simulink model "PthSet_TrqCalc"  (R2018a)
settings: configuration reference "cs_ert" (kept outside this file)
undefined symbols (not defined in the file): EngState, PthSet_trqOffs_C, TRQ_ZERO
libraries: simulink x4
settings Model: DataDictionary=PthSet_TrqCalc.sldd  Creator=zhoutinglin  LastModifiedBy=zhoutinglin

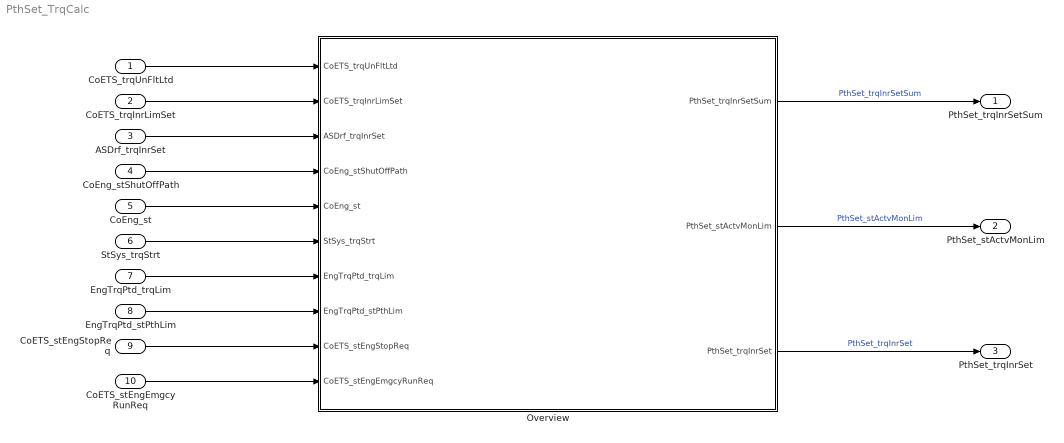
== system PthSet_TrqCalc ==
  CoETS_trqUnFltLtd : Inport  Description=Grip reliable exclude  OutMin=-3276  OutMax=3276  OutDataTypeStr=Torq  PortDimensions=[1 1]
  CoETS_trqInrLimSet : Inport  Description=Powertrain torque ratio  Port=2  OutMin=-3000  OutMax=3000  OutDataTypeStr=Torq  PortDimensions=[1 1]
  ASDrf_trqInrSet : Inport  Description=Limited idle speed governor torque  Port=3  OutMin=-3000  OutMax=3000  OutDataTypeStr=Torq  Unit=Nm  PortDimensions=[1 1]
  CoEng_stShutOffPath : Inport  Description=Limitation torque without the part of the speed governor  Port=4  OutMin=0  OutMax=65535  OutDataTypeStr=State2  PortDimensions=[1 1]
  CoEng_st : Inport  Description=ASD reference filter torque output  Port=5  OutDataTypeStr=Enum:EngState  PortDimensions=[1 1]
  StSys_trqStrt : Inport  Description=ASD disturbance compensator torque output  Port=6  OutMin=-3000  OutMax=3000  OutDataTypeStr=Torq  Unit=Nm  PortDimensions=[1 1]
  EngTrqPtd_trqLim : Inport  Description=Active shut-off paths resulting from active reversible,irreversible and afterrun shut-off paths  Port=7  OutMin=-3276  OutMax=3276  OutDataTypeStr=Torq  PortDimensions=[1 1]
  EngTrqPtd_stPthLim : Inport  Description=Engine coordinator state  Port=8  OutMin=0  OutMax=255  OutDataTypeStr=State  PortDimensions=[1 1]
  CoETS_stEngStopReq : Inport  Description=Engine starting torque  Port=9  OutMin=0  OutMax=1  OutDataTypeStr=boolean  PortDimensions=[1 1]
  CoETS_stEngEmgcyRunReq : Inport  Description=State of overrun detection (0: No overrun; 1: overrun)  Port=10  OutMin=0  OutMax=1  OutDataTypeStr=boolean  PortDimensions=[1 1]
  Overview : Subsystem
  PthSet_trqInrSetSum : Outport
  PthSet_stActvMonLim : Outport  Port=2
  PthSet_trqInrSet : Outport  Port=3
  wires:
  CoETS_trqUnFltLtd/1 -> Overview/1(CoETS_trqUnFltLtd)
  CoETS_trqInrLimSet/1 -> Overview/2(CoETS_trqInrLimSet)
  ASDrf_trqInrSet/1 -> Overview/3(ASDrf_trqInrSet)
  CoEng_stShutOffPath/1 -> Overview/4(CoEng_stShutOffPath)
  CoEng_st/1 -> Overview/5(CoEng_st)
  StSys_trqStrt/1 -> Overview/6(StSys_trqStrt)
  EngTrqPtd_trqLim/1 -> Overview/7(EngTrqPtd_trqLim)
  EngTrqPtd_stPthLim/1 -> Overview/8(EngTrqPtd_stPthLim)
  CoETS_stEngStopReq/1 -> Overview/9(CoETS_stEngStopReq)
  CoETS_stEngEmgcyRunReq/1 -> Overview/10(CoETS_stEngEmgcyRunReq)
  Overview/1(PthSet_trqInrSetSum) -> PthSet_trqInrSetSum/1  "PthSet_trqInrSetSum"
  Overview/2(PthSet_stActvMonLim) -> PthSet_stActvMonLim/1  "PthSet_stActvMonLim"
  Overview/3(PthSet_trqInrSet) -> PthSet_trqInrSet/1  "PthSet_trqInrSet"

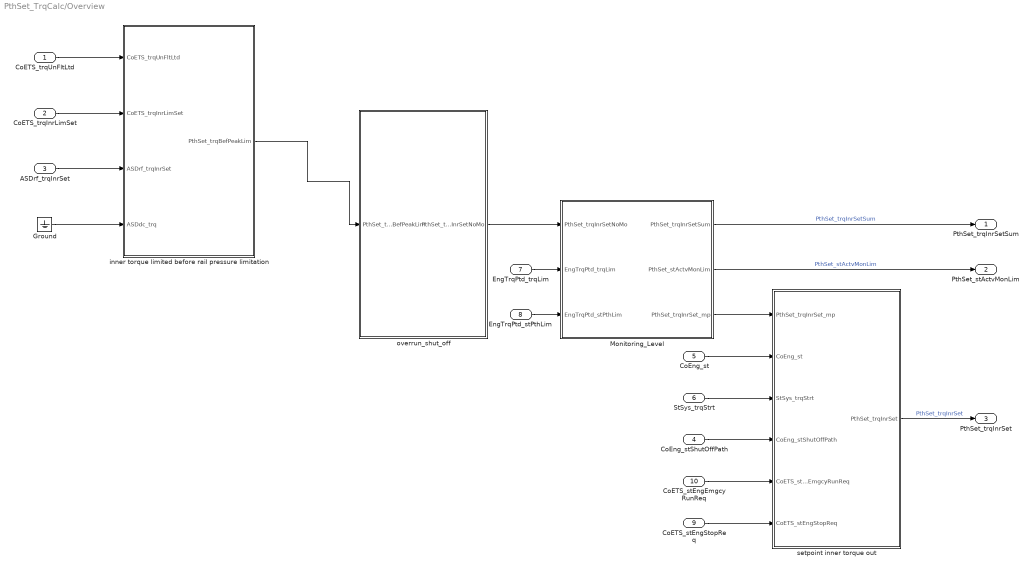
== system PthSet_TrqCalc/Overview ==
  CoETS_trqUnFltLtd : Inport  Tag=Nm
  CoETS_trqInrLimSet : Inport  Tag=Nm  Port=2
  ASDrf_trqInrSet : Inport  Tag=Nm  Port=3
  CoEng_stShutOffPath : Inport  Port=4
  CoEng_st : Inport  Port=5
  StSys_trqStrt : Inport  Tag=Nm  Port=6
  EngTrqPtd_trqLim : Inport  Tag=Nm  Port=7
  EngTrqPtd_stPthLim : Inport  Port=8
  CoETS_stEngStopReq : Inport  Port=9
  CoETS_stEngEmgcyRunReq : Inport  Port=10
  Ground : Ground
  Monitoring_Level : Subsystem
  inner torque limited before rail pressure limitation : Subsystem
  overrun_shut_off : Subsystem
  setpoint inner torque out : Subsystem
  PthSet_trqInrSetSum : Outport  Tag=Nm
  PthSet_stActvMonLim : Outport  Port=2
  PthSet_trqInrSet : Outport  Tag=Nm  Port=3
  wires:
  EngTrqPtd_trqLim/1 -> Monitoring_Level/2(EngTrqPtd_trqLim)
  CoETS_stEngStopReq/1 -> setpoint inner torque out/6(CoETS_stEngStopReq)
  inner torque limited before rail pressure limitation/1(PthSet_trqBefPeakLim) -> overrun_shut_off/1(PthSet_trqBefPeakLim)
  CoETS_trqInrLimSet/1 -> inner torque limited before rail pressure limitation/2(CoETS_trqInrLimSet)
  Monitoring_Level/3(PthSet_trqInrSet_mp) -> setpoint inner torque out/1(PthSet_trqInrSet_mp)
  Monitoring_Level/2(PthSet_stActvMonLim) -> PthSet_stActvMonLim/1  "PthSet_stActvMonLim"
  CoETS_trqUnFltLtd/1 -> inner torque limited before rail pressure limitation/1(CoETS_trqUnFltLtd)
  CoEng_stShutOffPath/1 -> setpoint inner torque out/4(CoEng_stShutOffPath)
  CoETS_stEngEmgcyRunReq/1 -> setpoint inner torque out/5(CoETS_stEngEmgcyRunReq)
  StSys_trqStrt/1 -> setpoint inner torque out/3(StSys_trqStrt)
  ASDrf_trqInrSet/1 -> inner torque limited before rail pressure limitation/3(ASDrf_trqInrSet)
  Monitoring_Level/1(PthSet_trqInrSetSum) -> PthSet_trqInrSetSum/1  "PthSet_trqInrSetSum"
  overrun_shut_off/1(PthSet_trqInrSetNoMo) -> Monitoring_Level/1(PthSet_trqInrSetNoMo)
  setpoint inner torque out/1(PthSet_trqInrSet) -> PthSet_trqInrSet/1  "PthSet_trqInrSet"
  CoEng_st/1 -> setpoint inner torque out/2(CoEng_st)
  Ground/1 -> inner torque limited before rail pressure limitation/4(ASDdc_trq)
  EngTrqPtd_stPthLim/1 -> Monitoring_Level/3(EngTrqPtd_stPthLim)

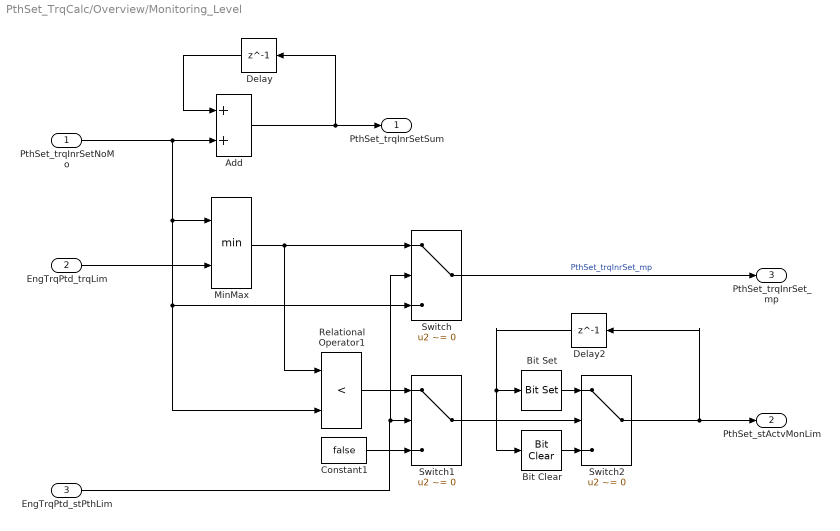
== system PthSet_TrqCalc/Overview/Monitoring_Level ==
  PthSet_trqInrSetNoMo : Inport
  EngTrqPtd_trqLim : Inport  Port=2
  EngTrqPtd_stPthLim : Inport  Port=3
  Add : Sum  SaturateOnIntegerOverflow=on  InputSameDT=on
  Bit Clear : simulink/Logic and Bit Operations/Bit Clear  iBit=0
      settings: SourceProductName=Simulink  SourceProductBaseCode=SL
  Bit Set : simulink/Logic and Bit Operations/Bit Set  iBit=0
      settings: SourceProductName=Simulink  SourceProductBaseCode=SL
  Constant1 : Constant  Value=false  OutDataTypeStr=Inherit: Inherit via back propagation
  Delay : Delay  DelayLength=1  InitialCondition=0
  Delay2 : Delay  DelayLength=1  InitialCondition=0
  MinMax : MinMax  Inputs=2  InputSameDT=on
  Relational Operator1 : RelationalOperator  Operator=<  OutDataTypeStr=boolean  RndMeth=Simplest  InputSameDT=on
  Switch : Switch  Criteria=u2 ~= 0  InputSameDT=on
  Switch1 : Switch  Criteria=u2 ~= 0  InputSameDT=on
  Switch2 : Switch  Criteria=u2 ~= 0  InputSameDT=on
  PthSet_trqInrSetSum : Outport
  PthSet_stActvMonLim : Outport  Port=2
  PthSet_trqInrSet_mp : Outport  Port=3
  wires:
  Delay2/1 -> Bit Set/1, Bit Clear/1
  Bit Clear/1 -> Switch2/3
  Bit Set/1 -> Switch2/1
  Switch2/1 -> PthSet_stActvMonLim/1, Delay2/1
  Switch1/1 -> Switch2/2
  Switch/1 -> PthSet_trqInrSet_mp/1  "PthSet_trqInrSet_mp"
  EngTrqPtd_stPthLim/1 -> Switch1/2, Switch/2
  Constant1/1 -> Switch1/3
  Relational Operator1/1 -> Switch1/1
  MinMax/1 -> Switch/1, Relational Operator1/1
  EngTrqPtd_trqLim/1 -> MinMax/2
  Delay/1 -> Add/1
  Add/1 -> PthSet_trqInrSetSum/1, Delay/1
  PthSet_trqInrSetNoMo/1 -> Add/2, MinMax/1, Switch/3, Relational Operator1/2

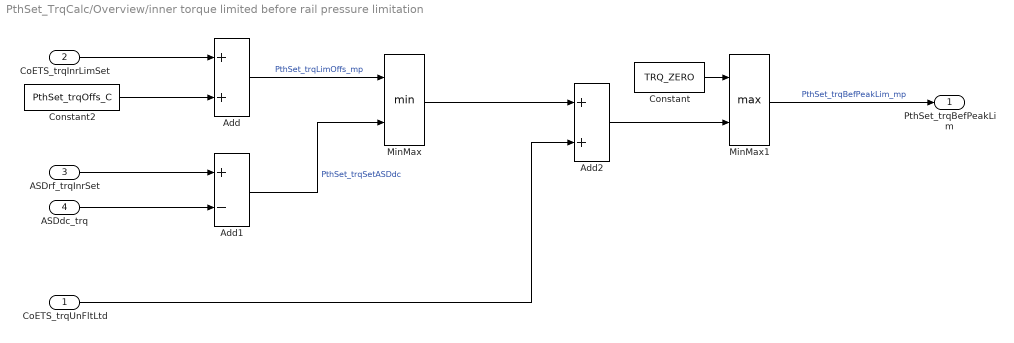
== system PthSet_TrqCalc/Overview/inner torque limited before rail pressure limitation ==
  CoETS_trqUnFltLtd : Inport
  CoETS_trqInrLimSet : Inport  Port=2
  ASDrf_trqInrSet : Inport  Port=3
  ASDdc_trq : Inport  Port=4
  Add : Sum  SaturateOnIntegerOverflow=on  InputSameDT=on
  Add1 : Sum  Inputs=+-  OutDataTypeStr=Inherit: Inherit via back propagation  SaturateOnIntegerOverflow=on  InputSameDT=on
  Add2 : Sum  SaturateOnIntegerOverflow=on  InputSameDT=on
  Constant : Constant  Value=TRQ_ZERO  OutDataTypeStr=Inherit: Inherit via back propagation
  Constant2 : Constant  Value=PthSet_trqOffs_C
  MinMax : MinMax  Inputs=2  InputSameDT=on
  MinMax1 : MinMax  Function=max  Inputs=2  InputSameDT=on
  PthSet_trqBefPeakLim : Outport
  wires:
  Constant2/1 -> Add/2
  ASDdc_trq/1 -> Add1/2
  Add2/1 -> MinMax1/2
  CoETS_trqInrLimSet/1 -> Add/1
  ASDrf_trqInrSet/1 -> Add1/1
  Add1/1 -> MinMax/2  "PthSet_trqSetASDdc"
  Add/1 -> MinMax/1  "PthSet_trqLimOffs_mp"
  CoETS_trqUnFltLtd/1 -> Add2/2
  MinMax/1 -> Add2/1
  Constant/1 -> MinMax1/1
  MinMax1/1 -> PthSet_trqBefPeakLim/1  "PthSet_trqBefPeakLim_mp"

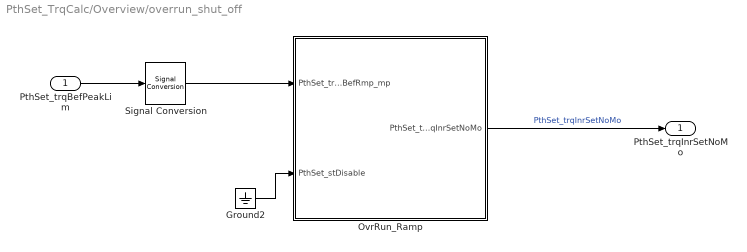
== system PthSet_TrqCalc/Overview/overrun_shut_off ==
  PthSet_trqBefPeakLim : Inport
  Ground2 : Ground
  OvrRun_Ramp : Subsystem
  Signal Conversion : SignalConversion  OverrideOpt=off
  PthSet_trqInrSetNoMo : Outport
  wires:
  PthSet_trqBefPeakLim/1 -> Signal Conversion/1
  Ground2/1 -> OvrRun_Ramp/2(PthSet_stDisable)
  OvrRun_Ramp/1(PthSet_trqInrSetNoMo) -> PthSet_trqInrSetNoMo/1  "PthSet_trqInrSetNoMo"
  Signal Conversion/1 -> OvrRun_Ramp/1(PthSet_trqBefRmp_mp)

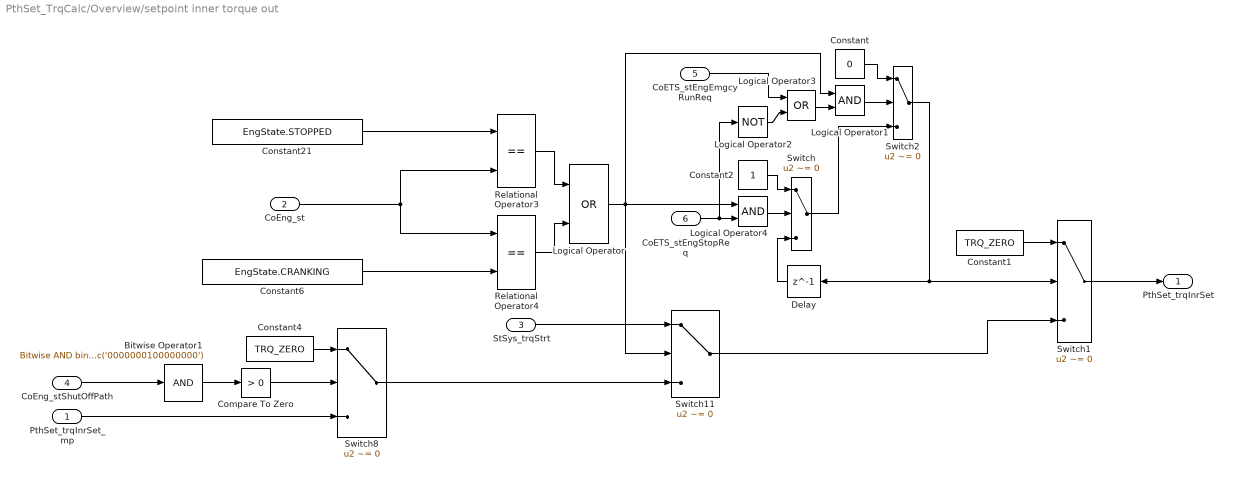
== system PthSet_TrqCalc/Overview/setpoint inner torque out ==
  PthSet_trqInrSet_mp : Inport
  CoEng_st : Inport  Port=2
  StSys_trqStrt : Inport  Port=3
  CoEng_stShutOffPath : Inport  Port=4
  CoETS_stEngEmgcyRunReq : Inport  Port=5
  CoETS_stEngStopReq : Inport  Port=6
  Bitwise Operator1 : simulink/Logic and Bit Operations/Bitwise Operator  logicop=AND  UseBitMask=on  BitMask=bin2dec('0000000100000000')  BitMaskRealWorld=Stored Integer
  Compare To Zero : simulink/Logic and Bit Operations/Compare To Zero  relop=>  OutDataTypeStr=boolean
  Constant : Constant  Value=0  OutDataTypeStr=Inherit: Inherit via back propagation
  Constant1 : Constant  Value=TRQ_ZERO  OutDataTypeStr=Inherit: Inherit via back propagation
  Constant2 : Constant  OutDataTypeStr=Inherit: Inherit via back propagation
  Constant21 : Constant  Value=EngState.STOPPED  OutDataTypeStr=Inherit: Inherit via back propagation
  Constant4 : Constant  Value=TRQ_ZERO  OutDataTypeStr=Inherit: Inherit via back propagation
  Constant6 : Constant  Value=EngState.CRANKING  OutDataTypeStr=Inherit: Inherit via back propagation
  Delay : Delay  DelayLength=1  InitialCondition=0
  Logical Operator : Logic  Operator=OR  OutDataTypeStr=boolean
  Logical Operator1 : Logic  AllPortsSameDT=off  OutDataTypeStr=boolean
  Logical Operator2 : Logic  Operator=NOT  AllPortsSameDT=off  OutDataTypeStr=boolean
  Logical Operator3 : Logic  Operator=OR  AllPortsSameDT=off  OutDataTypeStr=boolean
  Logical Operator4 : Logic  AllPortsSameDT=off  OutDataTypeStr=boolean
  Relational Operator3 : RelationalOperator  Operator===  OutDataTypeStr=boolean  RndMeth=Simplest  InputSameDT=on
  Relational Operator4 : RelationalOperator  Operator===  OutDataTypeStr=boolean  RndMeth=Simplest  InputSameDT=on
  Switch : Switch  Criteria=u2 ~= 0
  Switch1 : Switch  Criteria=u2 ~= 0  InputSameDT=on
  Switch11 : Switch  Criteria=u2 ~= 0  InputSameDT=on
  Switch2 : Switch  Criteria=u2 ~= 0
  Switch8 : Switch  Criteria=u2 ~= 0  InputSameDT=on
  PthSet_trqInrSet : Outport
  wires:
  Switch8/1 -> Switch11/3
  CoEng_st/1 -> Relational Operator3/2, Relational Operator4/1
  CoEng_stShutOffPath/1 -> Bitwise Operator1/1
  StSys_trqStrt/1 -> Switch11/1
  Constant6/1 -> Relational Operator4/2
  Constant21/1 -> Relational Operator3/1
  Constant4/1 -> Switch8/1
  Logical Operator/1 -> Logical Operator1/1, Logical Operator4/1, Switch11/2
  Relational Operator3/1 -> Logical Operator/1
  Relational Operator4/1 -> Logical Operator/2
  PthSet_trqInrSet_mp/1 -> Switch8/3
  Bitwise Operator1/1 -> Compare To Zero/1
  Compare To Zero/1 -> Switch8/2
  Switch11/1 -> Switch1/3
  Switch1/1 -> PthSet_trqInrSet/1
  Constant1/1 -> Switch1/1
  Switch2/1 -> Delay/1, Switch1/2
  Switch/1 -> Switch2/3
  Constant/1 -> Switch2/1
  Constant2/1 -> Switch/1
  Logical Operator1/1 -> Switch2/2
  Logical Operator2/1 -> Logical Operator3/2
  Logical Operator3/1 -> Logical Operator1/2
  CoETS_stEngEmgcyRunReq/1 -> Logical Operator3/1
  Logical Operator4/1 -> Switch/2
  CoETS_stEngStopReq/1 -> Logical Operator2/1, Logical Operator4/2
  Delay/1 -> Switch/3

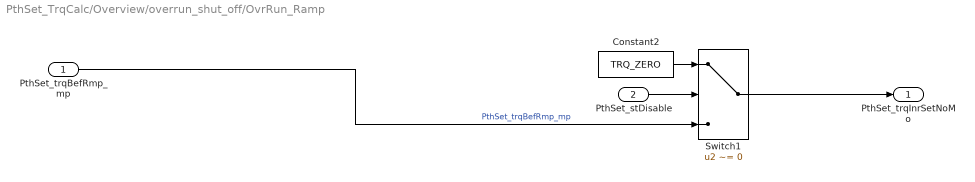
== system PthSet_TrqCalc/Overview/overrun_shut_off/OvrRun_Ramp ==
  PthSet_trqBefRmp_mp : Inport
  PthSet_stDisable : Inport  Port=2
  Constant2 : Constant  Value=TRQ_ZERO  OutDataTypeStr=Inherit: Inherit via back propagation
  Switch1 : Switch  Criteria=u2 ~= 0  InputSameDT=on
  PthSet_trqInrSetNoMo : Outport
  wires:
  PthSet_trqBefRmp_mp/1 -> Switch1/3  "PthSet_trqBefRmp_mp"
  Constant2/1 -> Switch1/1
  Switch1/1 -> PthSet_trqInrSetNoMo/1
  PthSet_stDisable/1 -> Switch1/2
